simulink model "Simu2"  (R2018b)
settings: Solver=VariableStepAuto  StartTime=0.0  StopTime=.02  RelTol=1e-3
values from neighbouring files (symbols this model uses):
  den2 = [L2*C2*R2 L2 R2]    [MainScript.m]
  num2 = [R2]    [MainScript.m]
settings Model: Creator=User  LastModifiedBy=charl
settings DebuggingCC: LibraryContextMissingDiagnostic=none
settings SFSimCC: SimUseLocalCustomCode=off
settings RTWCC: RTWUseLocalCustomCode=off

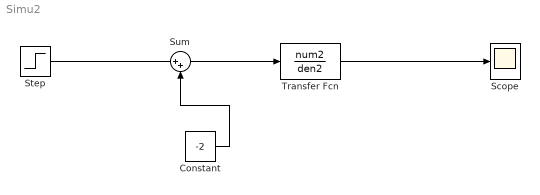
== system Simu2 ==
  Constant : Constant  Value=-2
  Scope : Scope
  Step : Step  Time=0  After=4  SampleTime=.00001  ZeroCross=off
  Sum : Sum  Inputs=|++
  Transfer Fcn : TransferFcn  Numerator=num2  Denominator=den2
  wires:
  Transfer Fcn/1 -> Scope/1
  Step/1 -> Transfer Fcn/1
  Constant/1 -> Sum/2
